simulink model "Red_problema6_Kclasica"  (R2021a)
settings: Solver=ode15s  StartTime=0.0  StopTime=sim_time  RelTol=1e-3
values from neighbouring files (symbols this model uses):
  aE112 = 177.25533427288616    (= 177.255334273)    [data_run_lazo_abierto_simulink.m]    (also in inicializar_areas.m = 179.376259805; script_IMC.m = a112_f)
  aE121 = 28.272251308900536    (= 28.2722513089)    [data_run_lazo_abierto_simulink.m]    (also in inicializar_areas.m; script_IMC.m = a121_f)
  aE213 = 304.960661680865    (= 304.960661681)    [data_run_lazo_abierto_simulink.m]    (also in inicializar_areas.m; script_IMC.m = a213_f)
  aE222 = 104.78323167686085    (= 104.783231677)    [data_run_lazo_abierto_simulink.m]    (also in inicializar_areas.m = 114.075570199; script_IMC.m = a222_f)
  aEcu1 = 2.44278466343862    (= 2.44278466344)    [data_run_lazo_abierto_simulink.m]    (also in inicializar_areas.m = 4.955447053)
  aEcu2 = 9.34130944614368    (= 9.34130944614)    [data_run_lazo_abierto_simulink.m]    (also in inicializar_areas.m = 18.78773145)
  aEhu2 = 53.1053199018638    (= 53.1053199019)    [data_run_lazo_abierto_simulink.m]    (also in inicializar_areas.m = 53.1053199)
  d1_end = 0    [data_run_lazo_abierto_simulink.m]    (also in inicializar_entradas.m; pert_max.m = 0.99; script_build_tfs.m)
  d1_in = 0    [data_run_lazo_abierto_simulink.m]    (also in inicializar_entradas.m; script_build_tfs.m)
  d2_end = 0    [data_run_lazo_abierto_simulink.m]    (also in inicializar_entradas.m; pert_max.m = 0.15; script_build_tfs.m)
  d2_in = 0    [data_run_lazo_abierto_simulink.m]    (also in inicializar_entradas.m; script_build_tfs.m)
  d3_end = 0    [data_run_lazo_abierto_simulink.m]    (also in inicializar_entradas.m; pert_max.m = 0.99; script_build_tfs.m)
  d3_in = 0    [data_run_lazo_abierto_simulink.m]    (also in inicializar_entradas.m; script_build_tfs.m)
  d4_end = 0    [data_run_lazo_abierto_simulink.m]    (also in inicializar_entradas.m; pert_max.m = 0.15; script_build_tfs.m)
  d4_in = 0    [data_run_lazo_abierto_simulink.m]    (also in inicializar_entradas.m; script_build_tfs.m)
  d5_end = 0    [data_run_lazo_abierto_simulink.m]    (also in inicializar_entradas.m; pert_max.m = -0.99; script_build_tfs.m)
  d5_in = 0    [data_run_lazo_abierto_simulink.m]    (also in inicializar_entradas.m; script_build_tfs.m)
  d6_end = 0    [data_run_lazo_abierto_simulink.m]    (also in inicializar_entradas.m; pert_max.m = 0.15; script_build_tfs.m)
  d6_in = 0    [data_run_lazo_abierto_simulink.m]    (also in inicializar_entradas.m; script_build_tfs.m)
  d7_end = 0    [data_run_lazo_abierto_simulink.m]    (also in inicializar_entradas.m; pert_max.m = -0.99; script_build_tfs.m)
  d7_in = 0    [data_run_lazo_abierto_simulink.m]    (also in inicializar_entradas.m; script_build_tfs.m)
  d8_end = 0    [data_run_lazo_abierto_simulink.m]    (also in inicializar_entradas.m; pert_max.m = 0.15; script_build_tfs.m)
  d8_in = 0    [data_run_lazo_abierto_simulink.m]    (also in inicializar_entradas.m; script_build_tfs.m)
  est = 1    [data_run_lazo_abierto_simulink.m]    (also in ini_comun.m; script_build_tfs.m)
  fc1 = 20    [data_run_lazo_abierto_simulink.m]    (also in ini_comun.m; script_build_tfs.m)
  fc2 = 50    [data_run_lazo_abierto_simulink.m]    (also in ini_comun.m; script_build_tfs.m)
  fcu1 = 36    [data_run_lazo_abierto_simulink.m]    (also in ini_comun.m = 1.45; inicializar_areas.m = 1.45; script_build_tfs.m = 1.45)
  fcu2 = 44    [data_run_lazo_abierto_simulink.m]    (also in ini_comun.m = 5; inicializar_areas.m = 5; script_build_tfs.m = 5)
  fh1 = 18    [data_run_lazo_abierto_simulink.m]    (also in ini_comun.m; script_build_tfs.m)
  fh2 = 22    [data_run_lazo_abierto_simulink.m]    (also in ini_comun.m; script_build_tfs.m)
  fhu2 = 14.8    [data_run_lazo_abierto_simulink.m]    (also in ini_comun.m = 15; inicializar_areas.m = 15; script_build_tfs.m = 15)
  hc1 = 1    [data_run_lazo_abierto_simulink.m]    (also in ini_comun.m; script_build_tfs.m)
  hc2 = 1    [data_run_lazo_abierto_simulink.m]    (also in ini_comun.m; script_build_tfs.m)
  hcu = 1    [data_run_lazo_abierto_simulink.m]    (also in ini_comun.m; script_build_tfs.m)
  hh1 = 1    [data_run_lazo_abierto_simulink.m]    (also in ini_comun.m; script_build_tfs.m)
  hh2 = 1    [data_run_lazo_abierto_simulink.m]    (also in ini_comun.m; script_build_tfs.m)
  hhu = 1    [data_run_lazo_abierto_simulink.m]    (also in ini_comun.m; script_build_tfs.m)
  initials = nominales_u_full    [cambiar_estructura.m]    (also in data_run_lazo_abierto_simulink.m; script_build_tfs.m)
  s1 = 30    [data_run_lazo_abierto_simulink.m]    (also in ini_comun.m; script_build_tfs.m)
  switch_var = 2    [script_IMC.m]
  t_step = 2000    [data_run_lazo_abierto_simulink.m]    (also in ini_comun.m = 20000; script_build_tfs.m = 1000)
  Tcin1 = 323    [data_run_lazo_abierto_simulink.m]    (also in ini_comun.m; script_build_tfs.m)
  Tcin2 = 433    [data_run_lazo_abierto_simulink.m]    (also in ini_comun.m; script_build_tfs.m)
  Tcuin = 288    [data_run_lazo_abierto_simulink.m]    (also in ini_comun.m; script_build_tfs.m)
  Thin1 = 543    [data_run_lazo_abierto_simulink.m]    (also in ini_comun.m; script_build_tfs.m)
  Thin2 = 493    [data_run_lazo_abierto_simulink.m]    (also in ini_comun.m; script_build_tfs.m)
  Thuin = 523    [data_run_lazo_abierto_simulink.m]    (also in ini_comun.m; script_build_tfs.m)
libraries: cstblocks x1, simulink x1
(part 2 of 2)

== system Red_problema6_Kclasica/Subsystem/inter_E112/valvula 3 ==
  In1 : Inport
  Gain : Gain  Gain=s1
  Gain1 : Gain  Gain=s1
  Integrator : Integrator
  Sum : Sum  Inputs=|+-
  Out1 : Outport  VectorParamsAs1DForOutWhenUnconnected=off
  wires:
  Gain1/1 -> Sum/2
  Integrator/1 -> Out1/1, Gain1/1
  Sum/1 -> Integrator/1
  Gain/1 -> Sum/1
  In1/1 -> Gain/1

== system Red_problema6_Kclasica/Subsystem/inter_E121/bypass ==
  note: la corriete 2 es la corriente del byapass
  note: la corriente 1 es la que se introduce al intercambiador
  1 : Inport
  u122 : Inport  Port=2
  Add : Sum  Inputs=+-
  Mux : Mux  Inputs=3
  Mux1 : Mux  Inputs=3
  Product : Product
  T : Fcn  Expr=u(1)
  f : Fcn  Expr=u(2)
  h : Fcn  Expr=u(3)
  " 1" : Outport  VectorParamsAs1DForOutWhenUnconnected=off
  " 2" : Outport  Port=2  VectorParamsAs1DForOutWhenUnconnected=off
  wires:
  u122/1 -> Product/1
  f/1 -> Add/1, Product/2
  Product/1 -> Mux1/2, Add/2
  1/1 -> T/1, h/1, f/1
  Add/1 -> Mux/2
  h/1 -> Mux1/3, Mux/3
  T/1 -> Mux1/1, Mux/1
  Mux/1 -> " 1"/1
  Mux1/1 -> " 2"/1

== system Red_problema6_Kclasica/Subsystem/inter_E121/bypass1 ==
  note: la corriente 1 es la que se introduce al intercambiador
  note: la corriete 2 es la corriente del byapass
  1 : Inport
  u122 : Inport  Port=2
  Add : Sum  Inputs=+-
  Mux : Mux  Inputs=3
  Mux1 : Mux  Inputs=3
  Product : Product
  T : Fcn  Expr=u(1)
  f : Fcn  Expr=u(2)
  h : Fcn  Expr=u(3)
  " 1" : Outport  VectorParamsAs1DForOutWhenUnconnected=off
  " 2" : Outport  Port=2  VectorParamsAs1DForOutWhenUnconnected=off
  wires:
  Mux1/1 -> " 2"/1
  Mux/1 -> " 1"/1
  T/1 -> Mux/1, Mux1/1
  h/1 -> Mux/3, Mux1/3
  Add/1 -> Mux/2
  1/1 -> f/1, h/1, T/1
  Product/1 -> Add/2, Mux1/2
  f/1 -> Product/2, Add/1
  u122/1 -> Product/1

== system Red_problema6_Kclasica/Subsystem/inter_E121/mux ==
  F1 : Inport
  F2 : Inport  Port=2
  Add : Sum
  Add1 : Sum
  Divide : Product  Inputs=*/
  Mux : Mux  Inputs=3
  Product : Product
  Product1 : Product
  T : Fcn  Expr=u(1)
  T1 : Fcn  Expr=u(1)
  Terminator : Terminator
  f : Fcn  Expr=u(2)
  f1 : Fcn  Expr=u(2)
  h : Fcn  Expr=u(3)
  h1 : Fcn  Expr=u(3)
  "F " : Outport  VectorParamsAs1DForOutWhenUnconnected=off
  wires:
  h/1 -> Mux/3
  Divide/1 -> Mux/1
  Add/1 -> Divide/2, Mux/2
  Add1/1 -> Divide/1
  Product1/1 -> Add1/2
  f1/1 -> Product1/2, Add/2
  T1/1 -> Product1/1
  Product/1 -> Add1/1
  T/1 -> Product/1
  F2/1 -> T1/1, f1/1, h1/1
  f/1 -> Add/1, Product/2
  F1/1 -> T/1, h/1, f/1
  Mux/1 -> "F "/1
  h1/1 -> Terminator/1

== system Red_problema6_Kclasica/Subsystem/inter_E121/mux1 ==
  F1 : Inport
  F2 : Inport  Port=2
  Add : Sum
  Add1 : Sum
  Divide : Product  Inputs=*/
  Mux : Mux  Inputs=3
  Product : Product
  Product1 : Product
  T : Fcn  Expr=u(1)
  T1 : Fcn  Expr=u(1)
  Terminator : Terminator
  f : Fcn  Expr=u(2)
  f1 : Fcn  Expr=u(2)
  h : Fcn  Expr=u(3)
  h1 : Fcn  Expr=u(3)
  "F " : Outport  VectorParamsAs1DForOutWhenUnconnected=off
  wires:
  Mux/1 -> "F "/1
  F1/1 -> f/1, h/1, T/1
  f/1 -> Product/2, Add/1
  F2/1 -> h1/1, f1/1, T1/1
  T/1 -> Product/1
  Product/1 -> Add1/1
  T1/1 -> Product1/1
  f1/1 -> Add/2, Product1/2
  Product1/1 -> Add1/2
  Add1/1 -> Divide/1
  Add/1 -> Mux/2, Divide/2
  Divide/1 -> Mux/1
  h/1 -> Mux/3
  h1/1 -> Terminator/1

== system Red_problema6_Kclasica/Subsystem/inter_E121/valvula 1 ==
  In1 : Inport
  Gain : Gain  Gain=s1
  Gain1 : Gain  Gain=s1
  Integrator : Integrator
  Sum : Sum  Inputs=|+-
  Out1 : Outport  VectorParamsAs1DForOutWhenUnconnected=off
  wires:
  Gain1/1 -> Sum/2
  Integrator/1 -> Out1/1, Gain1/1
  Sum/1 -> Integrator/1
  Gain/1 -> Sum/1
  In1/1 -> Gain/1

== system Red_problema6_Kclasica/Subsystem/inter_E121/valvula 3 ==
  In1 : Inport
  Gain : Gain  Gain=s1
  Gain1 : Gain  Gain=s1
  Integrator : Integrator
  Sum : Sum  Inputs=|+-
  Out1 : Outport  VectorParamsAs1DForOutWhenUnconnected=off
  wires:
  Gain1/1 -> Sum/2
  Integrator/1 -> Out1/1, Gain1/1
  Sum/1 -> Integrator/1
  Gain/1 -> Sum/1
  In1/1 -> Gain/1

== system Red_problema6_Kclasica/Subsystem/inter_E213/bypass ==
  note: la corriente 1 es la que se introduce al intercambiador
  note: la corriete 2 es la corriente del byapass
  1 : Inport
  u122 : Inport  Port=2
  Add : Sum  Inputs=+-
  Mux : Mux  Inputs=3
  Mux1 : Mux  Inputs=3
  Product : Product
  T : Fcn  Expr=u(1)
  f : Fcn  Expr=u(2)
  h : Fcn  Expr=u(3)
  " 1" : Outport  VectorParamsAs1DForOutWhenUnconnected=off
  " 2" : Outport  Port=2  VectorParamsAs1DForOutWhenUnconnected=off
  wires:
  Mux1/1 -> " 2"/1
  Mux/1 -> " 1"/1
  T/1 -> Mux/1, Mux1/1
  h/1 -> Mux/3, Mux1/3
  Add/1 -> Mux/2
  1/1 -> f/1, h/1, T/1
  Product/1 -> Add/2, Mux1/2
  f/1 -> Product/2, Add/1
  u122/1 -> Product/1

== system Red_problema6_Kclasica/Subsystem/inter_E213/bypass1 ==
  note: la corriete 2 es la corriente del byapass
  note: la corriente 1 es la que se introduce al intercambiador
  1 : Inport
  u122 : Inport  Port=2
  Add : Sum  Inputs=+-
  Mux : Mux  Inputs=3
  Mux1 : Mux  Inputs=3
  Product : Product
  T : Fcn  Expr=u(1)
  f : Fcn  Expr=u(2)
  h : Fcn  Expr=u(3)
  " 1" : Outport  VectorParamsAs1DForOutWhenUnconnected=off
  " 2" : Outport  Port=2  VectorParamsAs1DForOutWhenUnconnected=off
  wires:
  u122/1 -> Product/1
  f/1 -> Add/1, Product/2
  Product/1 -> Mux1/2, Add/2
  1/1 -> T/1, h/1, f/1
  Add/1 -> Mux/2
  h/1 -> Mux1/3, Mux/3
  T/1 -> Mux1/1, Mux/1
  Mux/1 -> " 1"/1
  Mux1/1 -> " 2"/1

== system Red_problema6_Kclasica/Subsystem/inter_E213/mux ==
  F1 : Inport
  F2 : Inport  Port=2
  Add : Sum
  Add1 : Sum
  Divide : Product  Inputs=*/
  Mux : Mux  Inputs=3
  Product : Product
  Product1 : Product
  T : Fcn  Expr=u(1)
  T1 : Fcn  Expr=u(1)
  Terminator : Terminator
  f : Fcn  Expr=u(2)
  f1 : Fcn  Expr=u(2)
  h : Fcn  Expr=u(3)
  h1 : Fcn  Expr=u(3)
  "F " : Outport  VectorParamsAs1DForOutWhenUnconnected=off
  wires:
  Mux/1 -> "F "/1
  F1/1 -> f/1, h/1, T/1
  f/1 -> Product/2, Add/1
  F2/1 -> h1/1, f1/1, T1/1
  T/1 -> Product/1
  Product/1 -> Add1/1
  T1/1 -> Product1/1
  f1/1 -> Add/2, Product1/2
  Product1/1 -> Add1/2
  Add1/1 -> Divide/1
  Add/1 -> Mux/2, Divide/2
  Divide/1 -> Mux/1
  h/1 -> Mux/3
  h1/1 -> Terminator/1

== system Red_problema6_Kclasica/Subsystem/inter_E213/mux1 ==
  F1 : Inport
  F2 : Inport  Port=2
  Add : Sum
  Add1 : Sum
  Divide : Product  Inputs=*/
  Mux : Mux  Inputs=3
  Product : Product
  Product1 : Product
  T : Fcn  Expr=u(1)
  T1 : Fcn  Expr=u(1)
  f : Fcn  Expr=u(2)
  f1 : Fcn  Expr=u(2)
  h : Fcn  Expr=u(3)
  h1 : Fcn  Expr=u(3)
  "F " : Outport  VectorParamsAs1DForOutWhenUnconnected=off
  wires:
  h/1 -> Mux/3
  Divide/1 -> Mux/1
  Add/1 -> Divide/2, Mux/2
  Add1/1 -> Divide/1
  Product1/1 -> Add1/2
  f1/1 -> Product1/2, Add/2
  T1/1 -> Product1/1
  Product/1 -> Add1/1
  T/1 -> Product/1
  F2/1 -> T1/1, f1/1, h1/1
  f/1 -> Add/1, Product/2
  F1/1 -> T/1, h/1, f/1
  Mux/1 -> "F "/1

== system Red_problema6_Kclasica/Subsystem/inter_E213/valvula 1 ==
  In1 : Inport
  Gain : Gain  Gain=s1
  Gain1 : Gain  Gain=s1
  Integrator : Integrator
  Sum : Sum  Inputs=|+-
  Out1 : Outport  VectorParamsAs1DForOutWhenUnconnected=off
  wires:
  Gain1/1 -> Sum/2
  Integrator/1 -> Out1/1, Gain1/1
  Sum/1 -> Integrator/1
  Gain/1 -> Sum/1
  In1/1 -> Gain/1

== system Red_problema6_Kclasica/Subsystem/inter_E213/valvula 3 ==
  In1 : Inport
  Gain : Gain  Gain=s1
  Gain1 : Gain  Gain=s1
  Integrator : Integrator
  Sum : Sum  Inputs=|+-
  Out1 : Outport  VectorParamsAs1DForOutWhenUnconnected=off
  wires:
  Gain1/1 -> Sum/2
  Integrator/1 -> Out1/1, Gain1/1
  Sum/1 -> Integrator/1
  Gain/1 -> Sum/1
  In1/1 -> Gain/1

== system Red_problema6_Kclasica/Subsystem/inter_E222/bypass ==
  note: la corriente 1 es la que se introduce al intercambiador
  note: la corriete 2 es la corriente del byapass
  1 : Inport
  u122 : Inport  Port=2
  Add : Sum  Inputs=+-
  Mux : Mux  Inputs=3
  Mux1 : Mux  Inputs=3
  Product : Product
  T : Fcn  Expr=u(1)
  f : Fcn  Expr=u(2)
  h : Fcn  Expr=u(3)
  " 1" : Outport  VectorParamsAs1DForOutWhenUnconnected=off
  " 2" : Outport  Port=2  VectorParamsAs1DForOutWhenUnconnected=off
  wires:
  Mux1/1 -> " 2"/1
  Mux/1 -> " 1"/1
  T/1 -> Mux/1, Mux1/1
  h/1 -> Mux/3, Mux1/3
  Add/1 -> Mux/2
  1/1 -> f/1, h/1, T/1
  Product/1 -> Add/2, Mux1/2
  f/1 -> Product/2, Add/1
  u122/1 -> Product/1

== system Red_problema6_Kclasica/Subsystem/inter_E222/bypass1 ==
  note: la corriete 2 es la corriente del byapass
  note: la corriente 1 es la que se introduce al intercambiador
  1 : Inport
  u122 : Inport  Port=2
  Add : Sum  Inputs=+-
  Mux : Mux  Inputs=3
  Mux1 : Mux  Inputs=3
  Product : Product
  T : Fcn  Expr=u(1)
  f : Fcn  Expr=u(2)
  h : Fcn  Expr=u(3)
  " 1" : Outport  VectorParamsAs1DForOutWhenUnconnected=off
  " 2" : Outport  Port=2  VectorParamsAs1DForOutWhenUnconnected=off
  wires:
  u122/1 -> Product/1
  f/1 -> Add/1, Product/2
  Product/1 -> Mux1/2, Add/2
  1/1 -> T/1, h/1, f/1
  Add/1 -> Mux/2
  h/1 -> Mux1/3, Mux/3
  T/1 -> Mux1/1, Mux/1
  Mux/1 -> " 1"/1
  Mux1/1 -> " 2"/1

== system Red_problema6_Kclasica/Subsystem/inter_E222/mux ==
  F1 : Inport
  F2 : Inport  Port=2
  Add : Sum
  Add1 : Sum
  Divide : Product  Inputs=*/
  Mux : Mux  Inputs=3
  Product : Product
  Product1 : Product
  T : Fcn  Expr=u(1)
  T1 : Fcn  Expr=u(1)
  Terminator : Terminator
  f : Fcn  Expr=u(2)
  f1 : Fcn  Expr=u(2)
  h : Fcn  Expr=u(3)
  h1 : Fcn  Expr=u(3)
  "F " : Outport  VectorParamsAs1DForOutWhenUnconnected=off
  wires:
  Mux/1 -> "F "/1
  F1/1 -> f/1, h/1, T/1
  f/1 -> Product/2, Add/1
  F2/1 -> h1/1, f1/1, T1/1
  T/1 -> Product/1
  Product/1 -> Add1/1
  T1/1 -> Product1/1
  f1/1 -> Add/2, Product1/2
  Product1/1 -> Add1/2
  Add1/1 -> Divide/1
  Add/1 -> Mux/2, Divide/2
  Divide/1 -> Mux/1
  h/1 -> Mux/3
  h1/1 -> Terminator/1

== system Red_problema6_Kclasica/Subsystem/inter_E222/mux1 ==
  F1 : Inport
  F2 : Inport  Port=2
  Add : Sum
  Add1 : Sum
  Divide : Product  Inputs=*/
  Mux : Mux  Inputs=3
  Product : Product
  Product1 : Product
  T : Fcn  Expr=u(1)
  T1 : Fcn  Expr=u(1)
  f : Fcn  Expr=u(2)
  f1 : Fcn  Expr=u(2)
  h : Fcn  Expr=u(3)
  h1 : Fcn  Expr=u(3)
  "F " : Outport  VectorParamsAs1DForOutWhenUnconnected=off
  wires:
  h/1 -> Mux/3
  Divide/1 -> Mux/1
  Add/1 -> Divide/2, Mux/2
  Add1/1 -> Divide/1
  Product1/1 -> Add1/2
  f1/1 -> Product1/2, Add/2
  T1/1 -> Product1/1
  Product/1 -> Add1/1
  T/1 -> Product/1
  F2/1 -> T1/1, f1/1, h1/1
  f/1 -> Add/1, Product/2
  F1/1 -> T/1, h/1, f/1
  Mux/1 -> "F "/1

== system Red_problema6_Kclasica/Subsystem/inter_E222/valvula 1 ==
  In1 : Inport
  Gain : Gain  Gain=s1
  Gain1 : Gain  Gain=s1
  Integrator : Integrator
  Sum : Sum  Inputs=|+-
  Out1 : Outport  VectorParamsAs1DForOutWhenUnconnected=off
  wires:
  Gain1/1 -> Sum/2
  Integrator/1 -> Out1/1, Gain1/1
  Sum/1 -> Integrator/1
  Gain/1 -> Sum/1
  In1/1 -> Gain/1

== system Red_problema6_Kclasica/Subsystem/inter_E222/valvula 3 ==
  In1 : Inport
  Gain : Gain  Gain=s1
  Gain1 : Gain  Gain=s1
  Integrator : Integrator
  Sum : Sum  Inputs=|+-
  Out1 : Outport  VectorParamsAs1DForOutWhenUnconnected=off
  wires:
  Gain1/1 -> Sum/2
  Integrator/1 -> Out1/1, Gain1/1
  Sum/1 -> Integrator/1
  Gain/1 -> Sum/1
  In1/1 -> Gain/1

== system Red_problema6_Kclasica/Subsystem/inter_Ecu_1/bypass ==
  note: la corriente 1 es la que se introduce al intercambiador
  note: la corriete 2 es la corriente del byapass
  1 : Inport
  u122 : Inport  Port=2
  Add : Sum  Inputs=+-
  Mux : Mux  Inputs=3
  Mux1 : Mux  Inputs=3
  Product : Product
  T : Fcn  Expr=u(1)
  f : Fcn  Expr=u(2)
  h : Fcn  Expr=u(3)
  " 1" : Outport  VectorParamsAs1DForOutWhenUnconnected=off
  " 2" : Outport  Port=2  VectorParamsAs1DForOutWhenUnconnected=off
  wires:
  Mux1/1 -> " 2"/1
  Mux/1 -> " 1"/1
  T/1 -> Mux/1, Mux1/1
  h/1 -> Mux/3, Mux1/3
  Add/1 -> Mux/2
  1/1 -> f/1, h/1, T/1
  Product/1 -> Add/2, Mux1/2
  f/1 -> Product/2, Add/1
  u122/1 -> Product/1

== system Red_problema6_Kclasica/Subsystem/inter_Ecu_1/bypass1 ==
  note: la corriete 2 es la corriente del byapass
  note: la corriente 1 es la que se introduce al intercambiador
  1 : Inport
  u122 : Inport  Port=2
  Add : Sum  Inputs=+-
  Mux : Mux  Inputs=3
  Mux1 : Mux  Inputs=3
  Product : Product
  T : Fcn  Expr=u(1)
  f : Fcn  Expr=u(2)
  h : Fcn  Expr=u(3)
  " 1" : Outport  VectorParamsAs1DForOutWhenUnconnected=off
  " 2" : Outport  Port=2  VectorParamsAs1DForOutWhenUnconnected=off
  wires:
  u122/1 -> Product/1
  f/1 -> Add/1, Product/2
  Product/1 -> Mux1/2, Add/2
  1/1 -> T/1, h/1, f/1
  Add/1 -> Mux/2
  h/1 -> Mux1/3, Mux/3
  T/1 -> Mux1/1, Mux/1
  Mux/1 -> " 1"/1
  Mux1/1 -> " 2"/1

== system Red_problema6_Kclasica/Subsystem/inter_Ecu_1/mux ==
  F1 : Inport
  F2 : Inport  Port=2
  Add : Sum
  Add1 : Sum
  Divide : Product  Inputs=*/
  Mux : Mux  Inputs=3
  Product : Product
  Product1 : Product
  T : Fcn  Expr=u(1)
  T1 : Fcn  Expr=u(1)
  Terminator : Terminator
  f : Fcn  Expr=u(2)
  f1 : Fcn  Expr=u(2)
  h : Fcn  Expr=u(3)
  h1 : Fcn  Expr=u(3)
  "F " : Outport  VectorParamsAs1DForOutWhenUnconnected=off
  wires:
  Mux/1 -> "F "/1
  F1/1 -> f/1, h/1, T/1
  f/1 -> Product/2, Add/1
  F2/1 -> h1/1, f1/1, T1/1
  T/1 -> Product/1
  Product/1 -> Add1/1
  T1/1 -> Product1/1
  f1/1 -> Add/2, Product1/2
  Product1/1 -> Add1/2
  Add1/1 -> Divide/1
  Add/1 -> Mux/2, Divide/2
  Divide/1 -> Mux/1
  h/1 -> Mux/3
  h1/1 -> Terminator/1

== system Red_problema6_Kclasica/Subsystem/inter_Ecu_1/mux1 ==
  F1 : Inport
  F2 : Inport  Port=2
  Add : Sum
  Add1 : Sum
  Divide : Product  Inputs=*/
  Mux : Mux  Inputs=3
  Product : Product
  Product1 : Product
  T : Fcn  Expr=u(1)
  T1 : Fcn  Expr=u(1)
  f : Fcn  Expr=u(2)
  f1 : Fcn  Expr=u(2)
  h : Fcn  Expr=u(3)
  h1 : Fcn  Expr=u(3)
  "F " : Outport  VectorParamsAs1DForOutWhenUnconnected=off
  wires:
  h/1 -> Mux/3
  Divide/1 -> Mux/1
  Add/1 -> Divide/2, Mux/2
  Add1/1 -> Divide/1
  Product1/1 -> Add1/2
  f1/1 -> Product1/2, Add/2
  T1/1 -> Product1/1
  Product/1 -> Add1/1
  T/1 -> Product/1
  F2/1 -> T1/1, f1/1, h1/1
  f/1 -> Add/1, Product/2
  F1/1 -> T/1, h/1, f/1
  Mux/1 -> "F "/1

== system Red_problema6_Kclasica/Subsystem/inter_Ecu_1/valvula 1 ==
  In1 : Inport
  Gain : Gain  Gain=s1
  Gain1 : Gain  Gain=s1
  Integrator : Integrator
  Sum : Sum  Inputs=|+-
  Out1 : Outport  VectorParamsAs1DForOutWhenUnconnected=off
  wires:
  Gain1/1 -> Sum/2
  Integrator/1 -> Out1/1, Gain1/1
  Sum/1 -> Integrator/1
  Gain/1 -> Sum/1
  In1/1 -> Gain/1

== system Red_problema6_Kclasica/Subsystem/inter_Ecu_1/valvula 3 ==
  In1 : Inport
  Gain : Gain  Gain=s1
  Gain1 : Gain  Gain=s1
  Integrator : Integrator
  Sum : Sum  Inputs=|+-
  Out1 : Outport  VectorParamsAs1DForOutWhenUnconnected=off
  wires:
  Gain1/1 -> Sum/2
  Integrator/1 -> Out1/1, Gain1/1
  Sum/1 -> Integrator/1
  Gain/1 -> Sum/1
  In1/1 -> Gain/1

== system Red_problema6_Kclasica/Subsystem/inter_Ecu_2/bypass ==
  note: la corriente 1 es la que se introduce al intercambiador
  note: la corriete 2 es la corriente del byapass
  1 : Inport
  u122 : Inport  Port=2
  Add : Sum  Inputs=+-
  Mux : Mux  Inputs=3
  Mux1 : Mux  Inputs=3
  Product : Product
  T : Fcn  Expr=u(1)
  f : Fcn  Expr=u(2)
  h : Fcn  Expr=u(3)
  " 1" : Outport  VectorParamsAs1DForOutWhenUnconnected=off
  " 2" : Outport  Port=2  VectorParamsAs1DForOutWhenUnconnected=off
  wires:
  Mux1/1 -> " 2"/1
  Mux/1 -> " 1"/1
  T/1 -> Mux/1, Mux1/1
  h/1 -> Mux/3, Mux1/3
  Add/1 -> Mux/2
  1/1 -> f/1, h/1, T/1
  Product/1 -> Add/2, Mux1/2
  f/1 -> Product/2, Add/1
  u122/1 -> Product/1

== system Red_problema6_Kclasica/Subsystem/inter_Ecu_2/bypass1 ==
  note: la corriete 2 es la corriente del byapass
  note: la corriente 1 es la que se introduce al intercambiador
  1 : Inport
  u122 : Inport  Port=2
  Add : Sum  Inputs=+-
  Mux : Mux  Inputs=3
  Mux1 : Mux  Inputs=3
  Product : Product
  T : Fcn  Expr=u(1)
  f : Fcn  Expr=u(2)
  h : Fcn  Expr=u(3)
  " 1" : Outport  VectorParamsAs1DForOutWhenUnconnected=off
  " 2" : Outport  Port=2  VectorParamsAs1DForOutWhenUnconnected=off
  wires:
  u122/1 -> Product/1
  f/1 -> Add/1, Product/2
  Product/1 -> Mux1/2, Add/2
  1/1 -> T/1, h/1, f/1
  Add/1 -> Mux/2
  h/1 -> Mux1/3, Mux/3
  T/1 -> Mux1/1, Mux/1
  Mux/1 -> " 1"/1
  Mux1/1 -> " 2"/1

== system Red_problema6_Kclasica/Subsystem/inter_Ecu_2/mux ==
  F1 : Inport
  F2 : Inport  Port=2
  Add : Sum
  Add1 : Sum
  Divide : Product  Inputs=*/
  Mux : Mux  Inputs=3
  Product : Product
  Product1 : Product
  T : Fcn  Expr=u(1)
  T1 : Fcn  Expr=u(1)
  Terminator : Terminator
  f : Fcn  Expr=u(2)
  f1 : Fcn  Expr=u(2)
  h : Fcn  Expr=u(3)
  h1 : Fcn  Expr=u(3)
  "F " : Outport  VectorParamsAs1DForOutWhenUnconnected=off
  wires:
  Mux/1 -> "F "/1
  F1/1 -> f/1, h/1, T/1
  f/1 -> Product/2, Add/1
  F2/1 -> h1/1, f1/1, T1/1
  T/1 -> Product/1
  Product/1 -> Add1/1
  T1/1 -> Product1/1
  f1/1 -> Add/2, Product1/2
  Product1/1 -> Add1/2
  Add1/1 -> Divide/1
  Add/1 -> Mux/2, Divide/2
  Divide/1 -> Mux/1
  h/1 -> Mux/3
  h1/1 -> Terminator/1

== system Red_problema6_Kclasica/Subsystem/inter_Ecu_2/mux1 ==
  F1 : Inport
  F2 : Inport  Port=2
  Add : Sum
  Add1 : Sum
  Divide : Product  Inputs=*/
  Mux : Mux  Inputs=3
  Product : Product
  Product1 : Product
  T : Fcn  Expr=u(1)
  T1 : Fcn  Expr=u(1)
  f : Fcn  Expr=u(2)
  f1 : Fcn  Expr=u(2)
  h : Fcn  Expr=u(3)
  h1 : Fcn  Expr=u(3)
  "F " : Outport  VectorParamsAs1DForOutWhenUnconnected=off
  wires:
  h/1 -> Mux/3
  Divide/1 -> Mux/1
  Add/1 -> Divide/2, Mux/2
  Add1/1 -> Divide/1
  Product1/1 -> Add1/2
  f1/1 -> Product1/2, Add/2
  T1/1 -> Product1/1
  Product/1 -> Add1/1
  T/1 -> Product/1
  F2/1 -> T1/1, f1/1, h1/1
  f/1 -> Add/1, Product/2
  F1/1 -> T/1, h/1, f/1
  Mux/1 -> "F "/1

== system Red_problema6_Kclasica/Subsystem/inter_Ecu_2/valvula 1 ==
  In1 : Inport
  Gain : Gain  Gain=s1
  Gain1 : Gain  Gain=s1
  Integrator : Integrator
  Sum : Sum  Inputs=|+-
  Out1 : Outport  VectorParamsAs1DForOutWhenUnconnected=off
  wires:
  Gain1/1 -> Sum/2
  Integrator/1 -> Out1/1, Gain1/1
  Sum/1 -> Integrator/1
  Gain/1 -> Sum/1
  In1/1 -> Gain/1

== system Red_problema6_Kclasica/Subsystem/inter_Ecu_2/valvula 3 ==
  In1 : Inport
  Gain : Gain  Gain=s1
  Gain1 : Gain  Gain=s1
  Integrator : Integrator
  Sum : Sum  Inputs=|+-
  Out1 : Outport  VectorParamsAs1DForOutWhenUnconnected=off
  wires:
  Gain1/1 -> Sum/2
  Integrator/1 -> Out1/1, Gain1/1
  Sum/1 -> Integrator/1
  Gain/1 -> Sum/1
  In1/1 -> Gain/1

== system Red_problema6_Kclasica/Subsystem/inter_Ehu_2/bypass ==
  note: la corriente 1 es la que se introduce al intercambiador
  note: la corriete 2 es la corriente del byapass
  1 : Inport
  u122 : Inport  Port=2
  Add : Sum  Inputs=+-
  Mux : Mux  Inputs=3
  Mux1 : Mux  Inputs=3
  Product : Product
  T : Fcn  Expr=u(1)
  f : Fcn  Expr=u(2)
  h : Fcn  Expr=u(3)
  " 1" : Outport  VectorParamsAs1DForOutWhenUnconnected=off
  " 2" : Outport  Port=2  VectorParamsAs1DForOutWhenUnconnected=off
  wires:
  Mux1/1 -> " 2"/1
  Mux/1 -> " 1"/1
  T/1 -> Mux/1, Mux1/1
  h/1 -> Mux/3, Mux1/3
  Add/1 -> Mux/2
  1/1 -> f/1, h/1, T/1
  Product/1 -> Add/2, Mux1/2
  f/1 -> Product/2, Add/1
  u122/1 -> Product/1

== system Red_problema6_Kclasica/Subsystem/inter_Ehu_2/bypass1 ==
  note: la corriete 2 es la corriente del byapass
  note: la corriente 1 es la que se introduce al intercambiador
  1 : Inport
  u122 : Inport  Port=2
  Add : Sum  Inputs=+-
  Mux : Mux  Inputs=3
  Mux1 : Mux  Inputs=3
  Product : Product
  T : Fcn  Expr=u(1)
  f : Fcn  Expr=u(2)
  h : Fcn  Expr=u(3)
  " 1" : Outport  VectorParamsAs1DForOutWhenUnconnected=off
  " 2" : Outport  Port=2  VectorParamsAs1DForOutWhenUnconnected=off
  wires:
  u122/1 -> Product/1
  f/1 -> Add/1, Product/2
  Product/1 -> Mux1/2, Add/2
  1/1 -> T/1, h/1, f/1
  Add/1 -> Mux/2
  h/1 -> Mux1/3, Mux/3
  T/1 -> Mux1/1, Mux/1
  Mux/1 -> " 1"/1
  Mux1/1 -> " 2"/1

== system Red_problema6_Kclasica/Subsystem/inter_Ehu_2/mux ==
  F1 : Inport
  F2 : Inport  Port=2
  Add : Sum
  Add1 : Sum
  Divide : Product  Inputs=*/
  Mux : Mux  Inputs=3
  Product : Product
  Product1 : Product
  T : Fcn  Expr=u(1)
  T1 : Fcn  Expr=u(1)
  Terminator : Terminator
  f : Fcn  Expr=u(2)
  f1 : Fcn  Expr=u(2)
  h : Fcn  Expr=u(3)
  h1 : Fcn  Expr=u(3)
  "F " : Outport  VectorParamsAs1DForOutWhenUnconnected=off
  wires:
  Mux/1 -> "F "/1
  F1/1 -> f/1, h/1, T/1
  f/1 -> Product/2, Add/1
  F2/1 -> h1/1, f1/1, T1/1
  T/1 -> Product/1
  Product/1 -> Add1/1
  T1/1 -> Product1/1
  f1/1 -> Add/2, Product1/2
  Product1/1 -> Add1/2
  Add1/1 -> Divide/1
  Add/1 -> Mux/2, Divide/2
  Divide/1 -> Mux/1
  h/1 -> Mux/3
  h1/1 -> Terminator/1

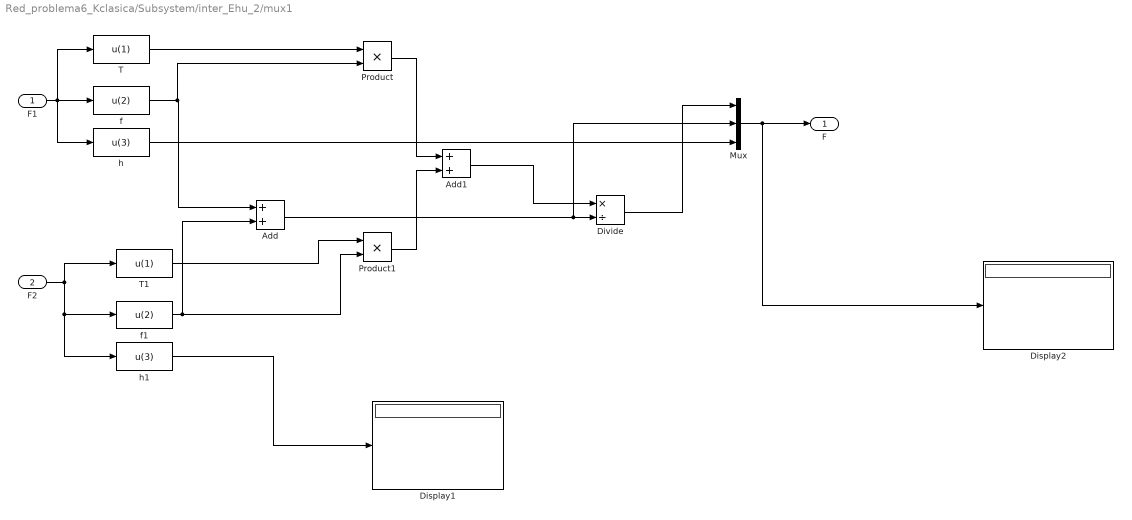
== system Red_problema6_Kclasica/Subsystem/inter_Ehu_2/mux1 ==
  F1 : Inport
  F2 : Inport  Port=2
  Add : Sum
  Add1 : Sum
  Display1 : Display
  Display2 : Display
  Divide : Product  Inputs=*/
  Mux : Mux  Inputs=3
  Product : Product
  Product1 : Product
  T : Fcn  Expr=u(1)
  T1 : Fcn  Expr=u(1)
  f : Fcn  Expr=u(2)
  f1 : Fcn  Expr=u(2)
  h : Fcn  Expr=u(3)
  h1 : Fcn  Expr=u(3)
  "F " : Outport  VectorParamsAs1DForOutWhenUnconnected=off
  wires:
  h/1 -> Mux/3
  Divide/1 -> Mux/1
  Add/1 -> Divide/2, Mux/2
  Add1/1 -> Divide/1
  Product1/1 -> Add1/2
  f1/1 -> Product1/2, Add/2
  T1/1 -> Product1/1
  Product/1 -> Add1/1
  T/1 -> Product/1
  F2/1 -> T1/1, f1/1, h1/1
  f/1 -> Add/1, Product/2
  F1/1 -> T/1, h/1, f/1
  Mux/1 -> Display2/1, "F "/1
  h1/1 -> Display1/1

== system Red_problema6_Kclasica/Subsystem/inter_Ehu_2/valvula 1 ==
  In1 : Inport
  Gain : Gain  Gain=s1
  Gain1 : Gain  Gain=s1
  Integrator : Integrator
  Sum : Sum  Inputs=|+-
  Out1 : Outport  VectorParamsAs1DForOutWhenUnconnected=off
  wires:
  Gain1/1 -> Sum/2
  Integrator/1 -> Out1/1, Gain1/1
  Sum/1 -> Integrator/1
  Gain/1 -> Sum/1
  In1/1 -> Gain/1

== system Red_problema6_Kclasica/Subsystem/inter_Ehu_2/valvula 3 ==
  In1 : Inport
  Gain : Gain  Gain=s1
  Gain1 : Gain  Gain=s1
  Integrator : Integrator
  Sum : Sum  Inputs=|+-
  Out1 : Outport  VectorParamsAs1DForOutWhenUnconnected=off
  wires:
  Gain1/1 -> Sum/2
  Integrator/1 -> Out1/1, Gain1/1
  Sum/1 -> Integrator/1
  Gain/1 -> Sum/1
  In1/1 -> Gain/1
